simulink model "Due_Fresh_model"  (R2020a)
settings: Solver=FixedStepAuto  StartTime=0.0  StopTime=inf  FixedStep=0.01  RelTol=1e-3  EnableMultiTasking=on
values from neighbouring files (symbols this model uses):
  Ad = sys_d.a    [fresh_code.m]
  Bd = sys_d.b    [fresh_code.m]
  Cd = sys_d.c    [fresh_code.m]
  Current_saturation = 2000    [fresh_code.m]
  Kd = dlqr(Ad,Bd,Q,R)    [fresh_code.m]
  Ld = place(Ad',Cd',Pd)'    [fresh_code.m]
  N_to_mAmp = 260    [fresh_code.m]
  Ndc = 1/dcgain(sys_d_cl(1))    [fresh_code.m]
  Ts = 1/100    (= 0.01)    [fresh_code.m]
libraries: arduinolib x3, etargetslib x2, simulink_extras x1, svdutilitieslib x1
settings Model: SILPILModeSetting=veronly  ExtModeTrigDuration=2  Creator=imkis  LastModifiedBy=imkis
settings OptimizationCC: DefaultUnderspecifiedDataType=single  EnhancedBackFolding=on  PassReuseOutputArgsAs=Individual arguments  ZeroExternalMemoryAtStartup=off  ZeroInternalMemoryAtStartup=off  MaxStackSize=64  OptimizeBlockOrder=speed  DifferentSizesBufferReuse=on  EfficientTunableParamExpr=on
settings DebuggingCC: ParameterPrecisionLossMsg=none  ParameterTunabilityLossMsg=error
settings HardwareCC: ProdBitPerPointer=32  ProdBitPerSizeT=32  ProdBitPerPtrDiffT=32  ProdLargestAtomicInteger=Long  ProdLargestAtomicFloat=Double  ProdWordSize=32  ProdHWDeviceType=ARM Compatible->ARM Cortex
settings SFSimCC: MATLABDynamicMemAlloc=off
settings RTWCC: SystemTargetFile=ert.tlc  HardwareBoard=Arduino Due  TLCOptions=-aInlineSetEventsForThisBaseRateFcn=TLC_FALSE -aSuppressMultiTaskScheduler=TLC_FALSE -aRateBasedStepFcn=1  TemplateMakefile=ert_default_tmf  Toolchain=Arduino ARM  BuildConfiguration=Faster Runs
settings CodeAppCC: ForceParamTrailComments=on  IgnoreCustomStorageClasses=off  OperatorAnnotations=on  SimulinkDataObjDesc=on  SFDataObjDesc=on  InsertBlockDesc=on
settings ERTTargetCC: SupportContinuousTime=on  SupportVariableSizeSignals=on  ExtModeStaticAllocSize=24576
settings ConfigComp: PLC_TargetIDE=codesys23

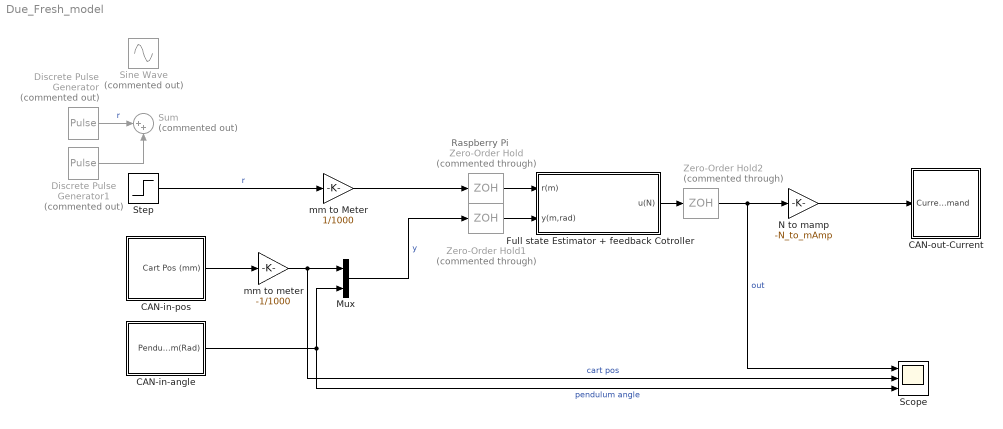
== system Due_Fresh_model ==
  note: Raspberry Pi
  CAN-in-angle : Subsystem
  CAN-in-pos : Subsystem
  CAN-out-Current : Subsystem
  Discrete Pulse Generator : DiscretePulseGenerator  Commented=on  Amplitude=100  Period=20/Ts  PulseWidth=5/Ts  PhaseDelay=10/Ts  SampleTime=Ts
  Discrete Pulse Generator1 : DiscretePulseGenerator  Commented=on  Amplitude=-100  Period=20/Ts  PulseWidth=5/Ts  PhaseDelay=20/Ts  SampleTime=Ts
  "Full state Estimator + feedback Cotroller " : Subsystem
  Mux : Mux  Inputs=2
  N to mamp : Gain  Gain=-N_to_mAmp
  Scope : Scope  NumInputPorts=3
  Sine Wave : Sin  Commented=on  Amplitude=100  Frequency=0.2*pi  Phase=10*pi  SampleTime=Ts
  Step : Step  Time=5  After=0  OutDataTypeStr=single  SampleTime=Ts
  Sum : Sum  Commented=on  Inputs=|++
  Zero-Order Hold : ZeroOrderHold  Commented=through  SampleTime=Ts
  Zero-Order Hold1 : ZeroOrderHold  Commented=through  SampleTime=Ts
  Zero-Order Hold2 : ZeroOrderHold  Commented=through  SampleTime=Ts
  mm to Meter : Gain  Gain=1/1000
  mm to meter : Gain  Gain=-1/1000
  wires:
  CAN-in-pos/1(Cart Pos (mm)) -> mm to meter/1
  CAN-in-angle/1(Pendulum(Rad)) -> Mux/2, Scope/3  "pendulum angle"
  mm to meter/1 -> Scope/2, Mux/1  "cart pos"
  N to mamp/1 -> CAN-out-Current/1("Current Command ")
  "Full state Estimator + feedback Cotroller "/1(u(N)) -> Zero-Order Hold2/1
  mm to Meter/1 -> Zero-Order Hold/1
  Mux/1 -> Zero-Order Hold1/1  "y"
  Zero-Order Hold/1 -> "Full state Estimator + feedback Cotroller "/1(r(m))
  Zero-Order Hold1/1 -> "Full state Estimator + feedback Cotroller "/2(y(m,rad))
  Zero-Order Hold2/1 -> Scope/1, N to mamp/1  "out"
  Step/1 -> mm to Meter/1  "r"
  Discrete Pulse Generator/1 -> Sum/1  "r"
  Discrete Pulse Generator1/1 -> Sum/2

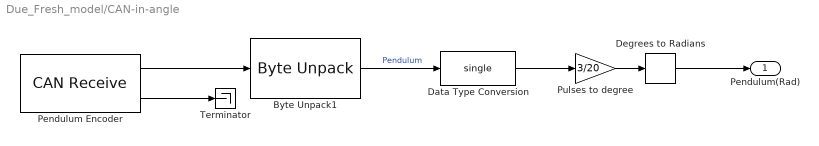
== system Due_Fresh_model/CAN-in-angle ==
  Byte Unpack1 : etargetslib/Byte Unpack  dimensions={[1]}  datatypes={'int32'}  byteAlign=4
  Data Type Conversion : DataTypeConversion  OutDataTypeStr=single
  Degrees to Radians : simulink_extras/Transformations/Degrees to Radians
  Pendulum Encoder : arduinolib/CAN Receive  outputDataType=Raw data  identifierType=Standard (11-bit identifier)  messageId=999  msgLength=4  SampleTime=Ts  outputError=off  outputRemote=off
      settings: SourceProductBaseCode=ARDUINO
  Pulses to degree : Gain  Gain=3/20
  Terminator : Terminator
  Pendulum(Rad) : Outport
  wires:
  Pendulum Encoder/2 -> Terminator/1
  Byte Unpack1/1 -> Data Type Conversion/1  "Pendulum"
  Pendulum Encoder/1 -> Byte Unpack1/1
  Pulses to degree/1 -> Degrees to Radians/1
  Degrees to Radians/1 -> Pendulum(Rad)/1
  Data Type Conversion/1 -> Pulses to degree/1

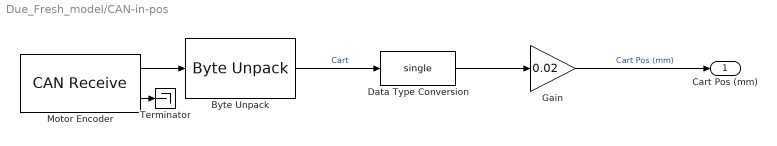
== system Due_Fresh_model/CAN-in-pos ==
  Byte Unpack : etargetslib/Byte Unpack  dimensions={[1]}  datatypes={'int32'}  byteAlign=4
  Data Type Conversion : DataTypeConversion  OutDataTypeStr=single
  Gain : Gain  Gain=0.02
  Motor Encoder : arduinolib/CAN Receive  outputDataType=Raw data  identifierType=Standard (11-bit identifier)  messageId=385  msgLength=4  SampleTime=Ts  outputError=off  outputRemote=off
      settings: SourceProductBaseCode=ARDUINO
  Terminator : Terminator
  Cart Pos (mm) : Outport
  wires:
  Byte Unpack/1 -> Data Type Conversion/1  "Cart"
  Motor Encoder/1 -> Byte Unpack/1
  Gain/1 -> Cart Pos (mm)/1  "Cart Pos (mm)"
  Motor Encoder/2 -> Terminator/1
  Data Type Conversion/1 -> Gain/1

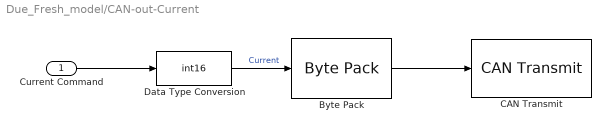
== system Due_Fresh_model/CAN-out-Current ==
  "Current Command " : Inport
  Byte Pack : svdutilitieslib/Byte Pack  maskPackedDataType=uint8  datatypes={'int16'}  byteAlign=2  blockPlatform=arduinoert
      settings: SourceProductBaseCode=ARDUINO,ML_ARDUINO,ECCORTEXA,ECCORTEXR,SC_BEAGLEBONE_BLUE,EC_FREEDOM_BOARD,EC_FRDM_K64F,INTEL_BLOCKSET,MICROBIT,NUCLEO,PX4AUTOPILOTS,RASPPIIO,STMICRODIS,TIC2000,XILINX_BLOCKSET
  CAN Transmit : arduinolib/CAN Transmit  inputDataType=Raw data  BlockingMode_=off  BlockTimeout_=1  outputStatus=off  identifierType=Standard (11-bit identifier)  messageId=hex2dec('201')  msgLength=2  remoteFrame=off
      settings: SourceProductBaseCode=ARDUINO
  Data Type Conversion : DataTypeConversion  OutDataTypeStr=int16
  wires:
  Data Type Conversion/1 -> Byte Pack/1  "Current"
  Byte Pack/1 -> CAN Transmit/1
  "Current Command "/1 -> Data Type Conversion/1

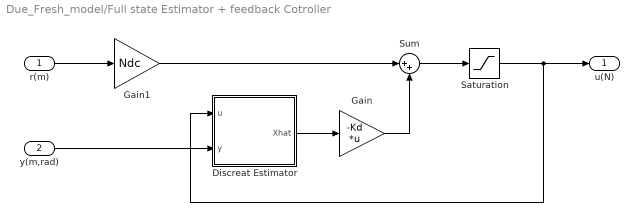
== system Due_Fresh_model/Full state Estimator + feedback Cotroller  ==
  r(m) : Inport
  y(m,rad) : Inport  Port=2
  Discreat Estimator : Subsystem
  Gain : Gain  Gain=-Kd  Multiplication=Matrix(K*u)
  Gain1 : Gain  Gain=Ndc
  Saturation : Saturate  UpperLimit=Current_saturation/N_to_mAmp  LowerLimit=-Current_saturation/N_to_mAmp
  Sum : Sum  Inputs=|++
  u(N) : Outport
  wires:
  Gain1/1 -> Sum/1
  Sum/1 -> Saturation/1
  y(m,rad)/1 -> Discreat Estimator/2(y)
  Discreat Estimator/1(Xhat) -> Gain/1
  Gain/1 -> Sum/2
  r(m)/1 -> Gain1/1
  Saturation/1 -> u(N)/1, Discreat Estimator/1(u)

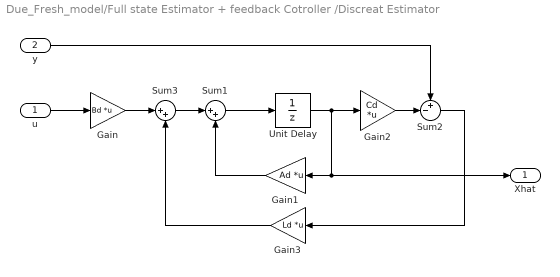
== system Due_Fresh_model/Full state Estimator + feedback Cotroller /Discreat Estimator ==
  u : Inport
  y : Inport  Port=2
  Gain : Gain  Gain=Bd  Multiplication=Matrix(K*u)
  Gain1 : Gain  Gain=Ad  Multiplication=Matrix(K*u)
  Gain2 : Gain  Gain=Cd  Multiplication=Matrix(K*u)
  Gain3 : Gain  Gain=Ld  Multiplication=Matrix(K*u)
  Sum1 : Sum  Inputs=|++
  Sum2 : Sum  Inputs=+-|
  Sum3 : Sum  Inputs=|++
  Unit Delay : UnitDelay  SampleTime=Ts  HasFrameUpgradeWarning=on
  Xhat : Outport
  wires:
  u/1 -> Gain/1
  y/1 -> Sum2/1
  Sum2/1 -> Gain3/1
  Sum1/1 -> Unit Delay/1
  Unit Delay/1 -> Xhat/1, Gain1/1, Gain2/1
  Gain2/1 -> Sum2/2
  Gain1/1 -> Sum1/2
  Gain3/1 -> Sum3/2
  Sum3/1 -> Sum1/1
  Gain/1 -> Sum3/1
